simulink model "simulare_regulator_discret_etapa2"  (R2020a)
settings: Solver=VariableStepAuto  StartTime=0.0  StopTime=500  RelTol=1e-3
settings Model: Creator=user  LastModifiedBy=user

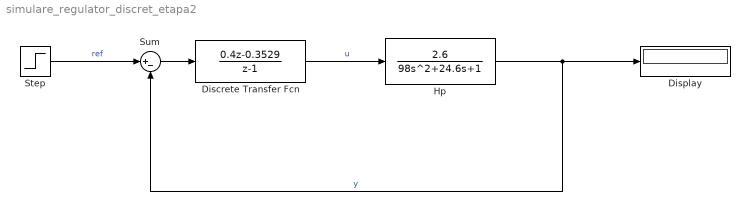
== system simulare_regulator_discret_etapa2 ==
  Discrete Transfer Fcn : DiscreteTransferFcn  Numerator=[0.4 -0.3529]  Denominator=[1 -1]  SampleTime=2.5
  Display : Display
  Hp : TransferFcn  Numerator=[2.6]  Denominator=[98 24.6 1]
  Step : Step  SampleTime=0
  Sum : Sum  Inputs=|+-
  wires:
  Hp/1 -> Display/1, Sum/2  "y"
  Step/1 -> Sum/1  "ref"
  Discrete Transfer Fcn/1 -> Hp/1  "u"
  Sum/1 -> Discrete Transfer Fcn/1
